simulink model "Q2_sim3"  (R2023b)
settings: Solver=VariableStepAuto  StartTime=0.0  StopTime=7  RelTol=1e-3
settings Model: Creator=avikd  LastModifiedBy=avikd

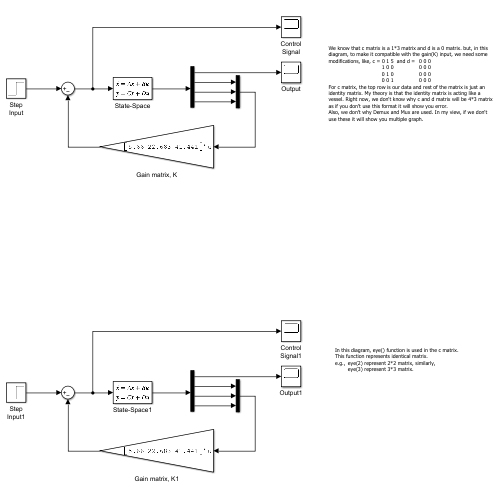
[thumbnail: Simulink's stored preview of the top-level diagram]
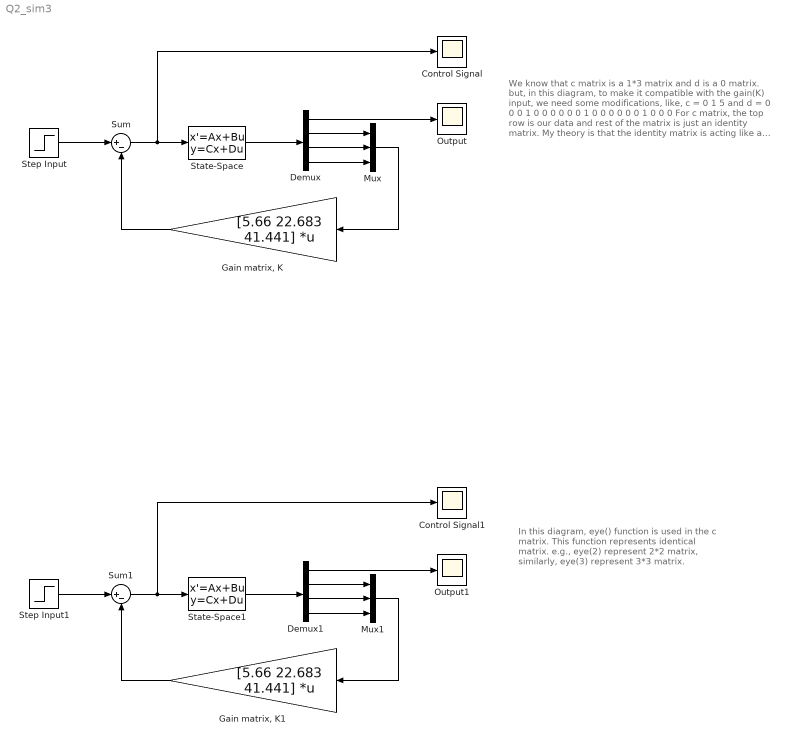
== system Q2_sim3 ==
  note: In this diagram, eye() function is used in the c matrix.
      | This function represents identical matrix.
      | e.g., eye(2) represent 2*2 matrix, similarly,
      | eye(3) represent 3*3 matrix.
  note: We know that c matrix is a 1*3 matrix and d is a 0 matrix. but, in this
      | diagram, to make it compatible with the gain(K) input, we need some
      | modifications, like, c = 0 1 5 and d = 0 0 0
      | 1 0 0 0 0 0
      | 0 1 0 0 0 0
      | 0 0 1 0 0 0
      | For c matrix, the top row is our data and rest of the matrix is just an
      | identity matrix. My theory is that the identity matrix is acting like a
      | vessel. Right now, we don't know why c and d matrix will be 4*3 matrix
      | as if you don't use this format it will show you error.
      | Also, we don't why Demux and Mux are used. In my view, if we don't
      | use these it will show you multiple graph.
  Control Signal : Scope
  Control Signal1 : Scope
  Demux : Demux
  Demux1 : Demux
  "Gain matrix, K" : Gain  Gain=[5.66 22.683 41.441]  Multiplication=Matrix(K*u)
  "Gain matrix, K1" : Gain  Gain=[5.66 22.683 41.441]  Multiplication=Matrix(K*u)
  Mux : Mux  Inputs=3
  Mux1 : Mux  Inputs=3
  Output : Scope
  Output1 : Scope
  State-Space : StateSpace  A=[-4 -1 6; 1 0 0; 0 1 0]  B=[1; 0; 0]  C=[0 1 5; 1 0 0; 0 1 0; 0 0 1]  D=[0; 0; 0; 0]  InitialCondition=0
  State-Space1 : StateSpace  A=[-4 -1 6; 1 0 0; 0 1 0]  B=[1; 0; 0]  C=[0 1 5; eye(3)]  D=[0; 0; 0; 0]  InitialCondition=0
  Step Input : Step  Time=0  SampleTime=0
  Step Input1 : Step  Time=0  SampleTime=0
  Sum : Sum  Inputs=|+-
  Sum1 : Sum  Inputs=|+-
  wires:
  Demux/1 -> Output/1
  Demux/2 -> Mux/1
  Demux/3 -> Mux/2
  Demux/4 -> Mux/3
  State-Space/1 -> Demux/1
  Step Input/1 -> Sum/1
  Sum/1 -> Control Signal/1, State-Space/1
  "Gain matrix, K"/1 -> Sum/2
  Mux/1 -> "Gain matrix, K"/1
  Demux1/2 -> Mux1/1
  Demux1/1 -> Output1/1
  Demux1/4 -> Mux1/3
  Mux1/1 -> "Gain matrix, K1"/1
  "Gain matrix, K1"/1 -> Sum1/2
  State-Space1/1 -> Demux1/1
  Sum1/1 -> Control Signal1/1, State-Space1/1
  Step Input1/1 -> Sum1/1
  Demux1/3 -> Mux1/2
